simulink model "Model_TranslationEngine64"  (R2022b)
settings: Solver=FixedStepDiscrete  StartTime=0.0  StopTime=5  RelTol=1e-3  EnableMultiTasking=on
InitFcn:
  | % Initialize model
  | ModelSettings=BTConfig.GetModelSettings();
  | 
  | ModelSettings.Validate();
  | 
  | ModelInit;
  | 
  | 
  | % load library data
  | GainLibrary_data;
  | % Load saved values from partition process
  | CapturedConstMask.LoadMapFromFile(bdroot)
StartFcn:
  | % make sure all the simulated RTC requests are found
  | %RTC_SIM_OBJ.ValidateREQs();
undefined symbols (not defined in the file or in its folder): AA, BPLP, Column, NumHFRefBPF, NumHFRefLPF, NumMusicChannels, Row, VolumeMuteConfig
libraries: TuneVar x925, TOP x490, FeaturePath x111, CapturedConstLib x52
(part 30 of 34)

== matlab function Model_TranslationEngine64/ModelPreAmp/DecRate/Medusa5H1/SleepingBeauty/SleepingBeauty/Enabled/FadeControl/InnerLink/TuneVarFadeTable/Fade_Table_Translation ==
  data: tableDb output; fadeTable input; tableIdx output
  events: trigger input FUNCTION_CALL_EVENT
function [tableDb, tableIdx] = fcn(fadeTable)
%#codegen

% Set up the size and datatype of our TOP outputs:
maxTableSize = numel(fadeTable.Value) / 2;
idxType = 'uint8';
idxStorageType = 'uint32';
dbType = 'single';
tableIdx = zeros(1,maxTableSize,idxStorageType);
tableDb = zeros(1,maxTableSize,dbType);

% separate the pairs into their index and value components
givenPairs = fadeTable.Size(1);
indexes = fadeTable.Value(1:givenPairs,1);
values = fadeTable.Value(1:givenPairs,2);

% then sort and ignore duplicates
[cleanIdx,map] = unique(indexes);

% Validate input sizes
numPairs = numel(map);
argName='FadeTable';

% Validate: enough data?
if (numPairs < 2)
    TranslateError('%s must have at least 2 index pairs. Encounted value with only %f pairs\n', argName, numPairs);
end

% Validate: Highest index still below 1.0?
if (cleanIdx(1) < 0 || cleanIdx(end) > intmax(idxType))
    TranslateError('%s out of range table index %f encountered. Index must be between 0 and 255.\n',argName,cleanIdx(end));
end

% fill in the table buffer with provided pairs
tableIdx(1:numPairs) = cleanIdx(1:numPairs);
tableDb(1:numPairs) = values(map(1:numPairs));

% fill the rest of the table buffer with the last entry
remainingPairs = numel(map)+1:maxTableSize;
tableIdx(remainingPairs) = tableIdx(numPairs);
tableDb(remainingPairs) =  tableDb(numPairs);

end

== matlab function Model_TranslationEngine64/ModelPreAmp/DecRate/Medusa5H1/SleepingBeauty/SleepingBeauty/Enabled/FadeRamperDR/InnerLink/Channel_Ramper_Translation ==
  data: ChanRampMap output; TuneChanRampMap input; channelCount input; MaskNumChannelGroups parameter
  events: trigger input FUNCTION_CALL_EVENT
function ChanRampMap  = fcn(TuneChanRampMap, channelCount,... % inputs
    MaskNumChannelGroups) % parameters

% Verifies if each channel is assigned to either the 'Front'(1) or 'Rear'(2)
% groups. 

argName = 'Fade';

% Ensure each channel is present in the map
inputMapWidth = numel(TuneChanRampMap.Value);
if (inputMapWidth ~= channelCount)
   error(['Error in %s : Channel-to-ramper map width [%d] does not match number of ',...
       'audio channels [%d]. Make sure all channels are assigned ',...
       'to either the front or rear groups.'], argName, inputMapWidth, ...
       channelCount);
end

% Verify that the channels are assigned to valid group numbers
if (numel(unique(TuneChanRampMap.Value)) > MaskNumChannelGroups + 1)
    error(['Error in [%s] : Atleast 1 channel has been assigned to an incorrect group. ' ...
        'Group numbers assigned to channels in the Channel-to-ramper '...
        'map should either be ''1'' (Front), ''2'' (Rear), or ''-1'' (Unused).'], argName);        
end

% Ensure that a value of 0 was not entered as a ramper
if (sum(TuneChanRampMap.Value == 0) > 0)
   error(['Error in [%s] : Valid ramper values for the channel to '...
       'ramper map must be either 1, 2, or "-1" to indicate an '... 
       'unused channel .'], argName);
end

% Output
ChanRampMap = int32(TuneChanRampMap.Value);

== matlab function Model_TranslationEngine64/ModelPreAmp/DecRate/Medusa5H1/MedusaHoligram/Medusa5H1 Part 3/On/VLS Gains Computation/VLS Gains Pax/SLC Tuning/Detent Level/Trivial Translation ==
  data: TOP output; detentGain input; configStruct parameter
  events: trigger input FUNCTION_CALL_EVENT
function TOP  = fcn(detentGain, configStruct)
%#codegen

% Checks if the parameter satisfies dimensionality requirements
if(detentGain.Size(1) ~= configStruct.numGains)
    TranslateError('The parameter ''VLS_gains_detent'' must be a %d element vector.', configStruct.numGains);
end

% Checks if the parameter values follow bound requirements
checkValues = (detentGain.Value < 0);    
if(sum(sum(checkValues)))       % Results in 0 if all values in the matrix respect the bound requirements
    TranslateError('The weights in ''VLS_gains_detent'' must be greater than or equal to 0.');
end

TOP = detentGain.Value;

end

== matlab function Model_TranslationEngine64/ModelPreAmp/DecRate/Medusa5H1/MedusaHoligram/Medusa5H1 Part 3/On/VLS Gains Computation/VLS Gains Pax/SLC Tuning/Interpolation Method/Trivial Translation ==
  data: TOP output; interpolationMethod input
  events: trigger input FUNCTION_CALL_EVENT
function TOP  = fcn(interpolationMethod)
%#codegen
% Checks if the parameter satisfies dimensionality requirements
if(numel(interpolationMethod.Value) ~= 1)
   TranslateError('The parameter ''medusa_surround_db_interpolation'' must be single dimensional.'); 
end

% Checks if the parameter value follows bound requirements
if((interpolationMethod.Value ~= 0) && (interpolationMethod.Value ~= 1))
   TranslateError('The value of ''medusa_surround_db_interpolation'' must be either 0 (for linear interpolation) or 1 (for dB-linear interpolation).'); 
end

TOP = interpolationMethod.Value;

end

== matlab function Model_TranslationEngine64/ModelPreAmp/DecRate/Medusa5H1/MedusaHoligram/Medusa5H1 Part 3/On/VLS Gains Computation/VLS Gains Pax/SLC Tuning/Max Level/Trivial Translation ==
  data: TOP output; maxGain input; configStruct parameter
  events: trigger input FUNCTION_CALL_EVENT
function TOP  = fcn(maxGain, configStruct)
%#codegen

% Checks if the parameter satisfies dimensionality requirements
if(maxGain.Size(1) ~= configStruct.numGains)
    TranslateError('The parameter ''VLS_gains_max'' must be a %d element vector.', configStruct.numGains);
end

% Checks if the parameter values follow bound requirements
checkValues = (maxGain.Value < 0);
if(sum(sum(checkValues)))          % Results in 0 if all values in the matrix respect the bound requirements
    TranslateError('The weights in ''VLS_gains_max'' must be greater than or equal to 0.');
end

TOP = maxGain.Value;

end

== matlab function Model_TranslationEngine64/ModelPreAmp/DecRate/Medusa5H1/MedusaHoligram/Medusa5H1 Part 3/On/VLS Gains Computation/VLS Gains Pax/SLC Tuning/Min Level/Trivial Translation ==
  data: TOP output; minGain input; configStruct parameter
  events: trigger input FUNCTION_CALL_EVENT
function TOP  = fcn(minGain, configStruct)
%#codegen

% Checks if the parameter satisfies dimensionality requirements
if(minGain.Size(1) ~= configStruct.numGains)
    TranslateError('The parameter ''VLS_gains_min'' must be a %d element vector.', configStruct.numGains);
end

% Checks if the parameter values follow bound requirements
checkValues = (minGain.Value < 0);
if(sum(sum(checkValues)))          % Results in 0 if all values in the matrix respect the bound requirements
    TranslateError('The weights in ''VLS_gains_min'' must be greater than or equal to 0.');
end

TOP = minGain.Value;

end

== matlab function Model_TranslationEngine64/ModelPreAmp/DecRate/Medusa5H1/SleepingBeauty/SleepingBeauty/Enabled/FadeRamperDR/InnerLink/Filter_Coeffs_Translation ==
  data: FilterCoeffs output; cutoffFreqHz input; FsHz input
  events: trigger input FUNCTION_CALL_EVENT
function FilterCoeffs  = fcn(cutoffFreqHz, FsHz)

% Generate the low pass filter coefficients which will then be applied to
% the audio input
% Inputs:
%  cutoffFreqHz: Cut off frequency in Hz for LPF
%  FsHz: Sampling frequency in Hz

omega = 2 * pi * cutoffFreqHz.Value / FsHz;

A = 1 - sin(omega) / cos(omega);
B0 = (1 - A) / 2;
B1 = B0;

FilterCoeffs = single([B0 B1 A]);

== matlab function Model_TranslationEngine64/ModelPreAmp/DecRate/Medusa5H1/SleepingBeauty/SleepingBeauty/Enabled/FadeRamperFR/InnerLink/Channel_Ramper_Translation ==
  data: ChanRampMap output; TuneChanRampMap input; channelCount input; MaskNumChannelGroups parameter
  events: trigger input FUNCTION_CALL_EVENT
function ChanRampMap  = fcn(TuneChanRampMap, channelCount,... % inputs
    MaskNumChannelGroups) % parameters

% Verifies if each channel is assigned to either the 'Front'(1) or 'Rear'(2)
% groups. 

argName = 'Fade';

% Ensure each channel is present in the map
inputMapWidth = numel(TuneChanRampMap.Value);
if (inputMapWidth ~= channelCount)
   error(['Error in %s : Channel-to-ramper map width [%d] does not match number of ',...
       'audio channels [%d]. Make sure all channels are assigned ',...
       'to either the front or rear groups.'], argName, inputMapWidth, ...
       channelCount);
end

% Verify that the channels are assigned to valid group numbers
if (numel(unique(TuneChanRampMap.Value)) > MaskNumChannelGroups + 1)
    error(['Error in [%s] : Atleast 1 channel has been assigned to an incorrect group. ' ...
        'Group numbers assigned to channels in the Channel-to-ramper '...
        'map should either be ''1'' (Front), ''2'' (Rear), or ''-1'' (Unused).'], argName);        
end

% Ensure that a value of 0 was not entered as a ramper
if (sum(TuneChanRampMap.Value == 0) > 0)
   error(['Error in [%s] : Valid ramper values for the channel to '...
       'ramper map must be either 1, 2, or "-1" to indicate an '... 
       'unused channel .'], argName);
end

% Output
ChanRampMap = int32(TuneChanRampMap.Value);

== matlab function Model_TranslationEngine64/ModelPreAmp/DecRate/Medusa5H1/SleepingBeauty/SleepingBeauty/Enabled/FadeRamperFR/InnerLink/Filter_Coeffs_Translation ==
  data: FilterCoeffs output; cutoffFreqHz input; FsHz input
  events: trigger input FUNCTION_CALL_EVENT
function FilterCoeffs  = fcn(cutoffFreqHz, FsHz)

% Generate the low pass filter coefficients which will then be applied to
% the audio input
% Inputs:
%  cutoffFreqHz: Cut off frequency in Hz for LPF
%  FsHz: Sampling frequency in Hz

omega = 2 * pi * cutoffFreqHz.Value / FsHz;

A = 1 - sin(omega) / cos(omega);
B0 = (1 - A) / 2;
B1 = B0;

FilterCoeffs = single([B0 B1 A]);

== matlab function Model_TranslationEngine64/ModelPreAmp/DecRate/AudioPilot35/EntertainmentLevelDetection/AudiopilotLevelDetect/AudiopilotLevelDetect/HoldMargin/SetPositive ==
  data: TOP output single; Tune input
  events: trigger input FUNCTION_CALL_EVENT
function TOP = fcn(Tune)
%#codegen

TOP = abs(Tune.Value);

== matlab function Model_TranslationEngine64/ModelPreAmp/DecRate/Medusa5H1/SleepingBeauty/SleepingBeauty/Enabled/SleepingBeautyFR/InnerLink/TuneVarTable/translation ==
  data: tableDb output; sleepingBeautyTable input; tableIdx output
  events: trigger input FUNCTION_CALL_EVENT
function [tableDb, tableIdx]  = fcn(sleepingBeautyTable)
%#codegen

% Set up the size and datatype of our TOP outputs:
maxTableSize = numel(sleepingBeautyTable.Value) / 2;
idxType = 'uint8';
idxStorageType = 'uint32';
dbType = 'single';
tableIdx = zeros(1,maxTableSize,idxStorageType);
tableDb = zeros(1,maxTableSize,dbType);

% separate the pairs into their index and value components
givenPairs = sleepingBeautyTable.Size(1);
indices = sleepingBeautyTable.Value(1:givenPairs,1);
values = sleepingBeautyTable.Value(1:givenPairs,2);

% then sort and ignore duplicates
[cleanIdx,map] = unique(indices);

% Validate input sizes
numPairs = numel(map);
argName='sleepingBeautyTable';

% Validate: enough data?
if (numPairs < 2)
    TranslateError('%s must have at least 2 index pairs. Encounted value with only %f pairs\n', argName, numPairs);
end

% Validate: Highest index still below 255?
if (cleanIdx(1) < 0 || cleanIdx(end) > intmax(idxType))
    TranslateError('%s out of range table index %f encountered. Index must be between 0 and %d.\n',argName,cleanIdx(end),intmax(idxType));
end

% fill in the table buffer with provided pairs
tableIdx(1:numPairs) = cleanIdx(1:numPairs);
tableDb(1:numPairs) = values(map(1:numPairs));

% fill the rest of the table buffer with the last entry
remainingPairs = numel(map)+1:maxTableSize;
tableIdx(remainingPairs) = tableIdx(numPairs);
tableDb(remainingPairs) =  tableDb(numPairs);

end

== matlab function Model_TranslationEngine64/ModelPreAmp/DecRate/Medusa5H1/VLS/VLS Generation - D/translation ==
  data: FIRCoeffs output; FIRCoeffsIn input; PaddedFIRLengthsIn input; PaddedFIRLengths output
  events: trigger input FUNCTION_CALL_EVENT
function [FIRCoeffs, PaddedFIRLengths] = fcn(FIRCoeffsIn, PaddedFIRLengthsIn)

FIRCoeffs = FIRCoeffsIn.Value;
PaddedFIRLengths = PaddedFIRLengthsIn.Value;

== matlab function Model_TranslationEngine64/ModelPreAmp/DecRate/Medusa5H1/SleepingBeauty/SleepingBeauty/Enabled/SleepingBeautyDR/InnerLink/channel_ramper_translation ==
  data: ChanRampMap output; TuneChanRampMap input; channelCount input; MaskNumRampers parameter
  events: trigger input FUNCTION_CALL_EVENT
function ChanRampMap = fcn(TuneChanRampMap, channelCount, ... %Inputs
    MaskNumRampers) % Parameters

% Function that verifies channel-to-ramper map is valid
% Takes channelRamperMap and channelCount as inputs, and 
% number of rampers as a parameter
argName = 'SleepingBeauty';

% Ensure each channel is present in the map
inputMapWidth = numel(TuneChanRampMap.Value);
if (inputMapWidth ~= channelCount)
   error(['Error in %s : Channel-to-ramper map width [%d] does not match number of ',...
       'audio channels [%d]. Make sure all channels are assigned ',...
       'to either the left or right groups.'], argName, inputMapWidth, ...
       channelCount);
end

% Verifies if each channel is assigned to one of the 5 possible rampers.

if (numel(unique(TuneChanRampMap.Value)) > (MaskNumRampers + 1))
    error(['Error in [%s] : Atleast 1 channel has been assigned to the incorrect group.' ...
        'Group numbers assigned to channels in the Channel-to-ramper '...
        'map should be a number between 1 and [%d], corresponding to one '...
        'of the 3 possible speaker contents .'], argName, MaskNumRampers);        
end

% Verify that a value of 0 was not incorrectly entered as a ramper
if (sum(TuneChanRampMap.Value == 0) > 0)
   error(['Error in [%s] : Valid ramper values for the channel to '...
       'ramper map must be between 1 and [%d}, or "-1" to indicate an '... 
       'unused channel .'], argName), MaskNumRampers;
end

ChanRampMap = int32(TuneChanRampMap.Value);

== matlab function Model_TranslationEngine64/ModelPreAmp/DecRate/Medusa5H1/VLS/Crosstalk Cancellation/Pooliir with Non-Trivial Translations/InnerLink/PoolIirTunableWithReset/Translation ==
  data: RawSOS input; NumStages input; PoolNumStages output; PoolCoeffs output; MaxNumStages parameter; VariantUint8 parameter; NumChannels input
  events: trigger input FUNCTION_CALL_EVENT
function [PoolNumStages, PoolCoeffs] = pooliirTranslation(RawSOS, NumStages, MaxNumStages, VariantUint8,  NumChannels)
%#codegen

% Translation from raw SOS for pool SOS

% Some build time sanity size checking before calling the translation
if numel(NumStages.Value) ~= NumChannels
    error('Size of num stages has to match number of input channels')
end

if RawSOS.Size(2) ~= 6
    error ('Coefficient pool matrix must have 6 columns')
end

[PoolNumStages, PoolCoeffs] = poolIirTranslation(RawSOS, NumStages, MaxNumStages, VariantUint8);

% VariantStr = char(VariantUint8);
% switch (VariantStr)
%     case {"Generic","SharcPlusCore"}
%         % These variants order biquad coefficients in a compacted form
%         [PoolNumStages, PoolCoeffs] = pooliirTranslationFcn(RawSOS, NumStages, MaxNumStages);
%     case {"SharcPlusAccelGul","SharcPlusAccelGxp"}
%         % These variants order biquad coefficients for the ADI accelerator
%         [PoolNumStages, PoolCoeffs] = pooliirAccelTranslationFcn(RawSOS, NumStages, MaxNumStages);
%     case{"Hexagon"}
%         % Hexagon specific order for biquad coefficients 
%         [PoolNumStages, PoolCoeffs] = PoolIirHexagonTranslationFcn(RawSOS, NumStages, MaxNumStages);
%     case{"ArmNeonV7V8"}
%         [PoolNumStages, PoolCoeffs] = PoolIirArmNeonV7V8TranslationFcn(RawSOS, NumStages, MaxNumStages);
%     otherwise
%         % This is a build-time error, not a translation error. The
%         % selected build-time variant is not supported for translation
%         error('Invalid implementation type: [%s]', VariantStr);
% end

end

== matlab function Model_TranslationEngine64/ModelPreAmp/DecRate/Medusa5H1/SleepingBeauty/SleepingBeauty/Enabled/SleepingBeautyFR/InnerLink/channel_ramper_translation ==
  data: ChanRampMap output; TuneChanRampMap input; channelCount input; MaskNumRampers parameter
  events: trigger input FUNCTION_CALL_EVENT
function ChanRampMap = fcn(TuneChanRampMap, channelCount, ... %Inputs
    MaskNumRampers) % Parameters

% Function that verifies channel-to-ramper map is valid
% Takes channelRamperMap and channelCount as inputs, and 
% number of rampers as a parameter
argName = 'SleepingBeauty';

% Ensure each channel is present in the map
inputMapWidth = numel(TuneChanRampMap.Value);
if (inputMapWidth ~= channelCount)
   error(['Error in %s : Channel-to-ramper map width [%d] does not match number of ',...
       'audio channels [%d]. Make sure all channels are assigned ',...
       'to either the left or right groups.'], argName, inputMapWidth, ...
       channelCount);
end

% Verifies if each channel is assigned to one of the 5 possible rampers.

if (numel(unique(TuneChanRampMap.Value)) > (MaskNumRampers + 1))
    error(['Error in [%s] : Atleast 1 channel has been assigned to the incorrect group.' ...
        'Group numbers assigned to channels in the Channel-to-ramper '...
        'map should be a number between 1 and [%d], corresponding to one '...
        'of the 3 possible speaker contents .'], argName, MaskNumRampers);        
end

% Verify that a value of 0 was not incorrectly entered as a ramper
if (sum(TuneChanRampMap.Value == 0) > 0)
   error(['Error in [%s] : Valid ramper values for the channel to '...
       'ramper map must be between 1 and [%d}, or "-1" to indicate an '... 
       'unused channel .'], argName), MaskNumRampers;
end

ChanRampMap = int32(TuneChanRampMap.Value);

== matlab function Model_TranslationEngine64/ModelPreAmp/DecRate/Medusa5H1/VLS/VLS Generation - P/translation ==
  data: FIRCoeffs output; FIRCoeffsIn input; PaddedFIRLengthsIn input; PaddedFIRLengths output
  events: trigger input FUNCTION_CALL_EVENT
function [FIRCoeffs, PaddedFIRLengths] = fcn(FIRCoeffsIn, PaddedFIRLengthsIn)

FIRCoeffs = FIRCoeffsIn.Value;
PaddedFIRLengths = PaddedFIRLengthsIn.Value;

== matlab function Model_TranslationEngine64/ModelPreAmp/PreAmpPart1/NEARPreAmp/FixedAttenuator/Attenuation /Function-Call Subsystem/MATLAB Function ==
  data: dbgain input; lingain output
function lingain = fcn(dbgain)
    lingain = 10^(dbgain.Value/20);   
end

== matlab function Model_TranslationEngine64/NEAR/Near1p1/VolumeMute/AnnouncementLevelDetector/ch1_level/fast_decay/sec2samples ==
  data: y output; u input; FrameRate parameter
  events: trigger input FUNCTION_CALL_EVENT
function y  = fcn(u,FrameRate)
%#codegen

y = -abs(u.Value/FrameRate);

== matlab function Model_TranslationEngine64/ModelPreAmp/DecRate/Medusa5H1/SleepingBeauty/SleepingBeauty/Enabled/SleepingBeautyDR/InnerLink/TuneVarTable/translation ==
  data: tableDb output; sleepingBeautyTable input; tableIdx output
  events: trigger input FUNCTION_CALL_EVENT
function [tableDb, tableIdx]  = fcn(sleepingBeautyTable)
%#codegen

% Set up the size and datatype of our TOP outputs:
maxTableSize = numel(sleepingBeautyTable.Value) / 2;
idxType = 'uint8';
idxStorageType = 'uint32';
dbType = 'single';
tableIdx = zeros(1,maxTableSize,idxStorageType);
tableDb = zeros(1,maxTableSize,dbType);

% separate the pairs into their index and value components
givenPairs = sleepingBeautyTable.Size(1);
indices = sleepingBeautyTable.Value(1:givenPairs,1);
values = sleepingBeautyTable.Value(1:givenPairs,2);

% then sort and ignore duplicates
[cleanIdx,map] = unique(indices);

% Validate input sizes
numPairs = numel(map);
argName='sleepingBeautyTable';

% Validate: enough data?
if (numPairs < 2)
    TranslateError('%s must have at least 2 index pairs. Encounted value with only %f pairs\n', argName, numPairs);
end

% Validate: Highest index still below 255?
if (cleanIdx(1) < 0 || cleanIdx(end) > intmax(idxType))
    TranslateError('%s out of range table index %f encountered. Index must be between 0 and %d.\n',argName,cleanIdx(end),intmax(idxType));
end

% fill in the table buffer with provided pairs
tableIdx(1:numPairs) = cleanIdx(1:numPairs);
tableDb(1:numPairs) = values(map(1:numPairs));

% fill the rest of the table buffer with the last entry
remainingPairs = numel(map)+1:maxTableSize;
tableIdx(remainingPairs) = tableIdx(numPairs);
tableDb(remainingPairs) =  tableDb(numPairs);

end

== matlab function Model_TranslationEngine64/NEAR/Near1p1/VolumeMute/AnnouncementLevelDetector/ch1_level/hold_margin/SetPositive ==
  data: TOP output single; Tune input
  events: trigger input FUNCTION_CALL_EVENT
function TOP = fcn(Tune)
%#codegen

TOP = abs(Tune.Value);

== matlab function Model_TranslationEngine64/ModelPreAmp/PreAmpPart1/NEARPreAmp/MusicLimiter/annPredTuneTOP/Trivial Translation ==
  data: TOP1 output; Tune1 input
  events: trigger input FUNCTION_CALL_EVENT
function TOP1  = fcn(Tune1)
%#codegen

% ----- To access TuneVar maximum size, current size, and current value:
%   Note: TuneVar signals arrive with exposed variable size information.
%         The expressions below illustrate for the "Tune1" input argument.
%
%   size(Tune1.Value) : the maximum possible size of the Tune1 variable
%
%   Tune.Size   : the current size of *valid* data in Tune1.Value
%
%   Tune1.Size(1) : Number of rows present in Tune1 - this does not vary.
%
%   Tune1.Size(2) : Number of columns currently valid in Tune1 - this is
%       the variable part of size that can change (if allowed by TuneVar).
%
%   Tune1.Value : the current value of the tune variable... but end-padded 
%       to the maximum available size with undefined/invalid data.
%
%   numel(Tune1.Value) : another way of looking at the maximum number of
%       elements that could arrive in Tune1.Value
%
% ----- To register an error, use the following method (works like printf):
%   TranslateError( <format string>, <arguments ... )
%   ... this error will cause the build process to abort.

% A trivial pass-through translation looks like this:
%TOP1 = Tune1.Value;
TOP1 = 10 ^ ((Tune1.Value) / 20);

== matlab function Model_TranslationEngine64/NEAR/Near1p1/VolumeMute/AnnouncementLevelDetector/ch1_level/hold_time/sec2samples ==
  data: y output; u input; FrameRate parameter
  events: trigger input FUNCTION_CALL_EVENT
function y  = fcn(u,FrameRate)
%#codegen

y = ceil(u.Value*FrameRate);

== matlab function Model_TranslationEngine64/ModelPreAmp/PreAmpPart1/Bass/tone filter tune translate1 ==
  data: FilterCoeffs output; FilterFrequencyHz input; Fs input; MaskFilterType parameter
  events: trigger input FUNCTION_CALL_EVENT
function FilterCoeffs  = fcn( ...
    FilterFrequencyHz, Fs, ... % inputs
    MaskFilterType ) % parameters
%#codegen

omega = 2 * pi * FilterFrequencyHz.Value / Fs;

A = (1 - sin(omega)) / cos(omega);

if (MaskFilterType == ToneMask.TypeLowpass)
    % lowpass coeffs (e.g. bass)
    B0 = (1 - A) / 2;
    B1 = B0;
else
    % highpass coeffs (e.g. treble)
    B0 = (1 + A) / 2;
    B1 = 0 - B0;
end

FilterCoeffs = single([B0 B1 A]);

== matlab function Model_TranslationEngine64/ModelPreAmp/PreAmpPart1/Bass/tone filter tune translate2 ==
  data: FilterCoeffs output; FilterFrequencyHz input; Fs input; MaskFilterType parameter
  events: trigger input FUNCTION_CALL_EVENT
function FilterCoeffs  = fcn( ...
    FilterFrequencyHz, Fs, ... % inputs
    MaskFilterType ) % parameters
%#codegen

omega = 2 * pi * FilterFrequencyHz.Value / Fs;

A = (1 - sin(omega)) / cos(omega);

if (MaskFilterType == ToneMask.TypeLowpass)
    % lowpass coeffs (e.g. bass)
    B0 = (1 - A) / 2;
    B1 = B0;
else
    % highpass coeffs (e.g. treble)
    B0 = (1 + A) / 2;
    B1 = 0 - B0;
end

FilterCoeffs = single([B0 B1 A]);

== matlab function Model_TranslationEngine64/ModelPreAmp/PreAmpPart1/Bass/tone filter tune translate3 ==
  data: maxOut output; maxIn input
  events: trigger input FUNCTION_CALL_EVENT
function maxOut  = fcn( ...
    maxIn) ... % inputs % parameters
%#codegen

% Just make sure the maximum is a positive dB value
maxOut = single(abs(maxIn.Value));

== matlab function Model_TranslationEngine64/ModelPreAmp/PreAmpPart1/Bass/tone filter tune translate4 ==
  data: maxOut output; maxIn input
  events: trigger input FUNCTION_CALL_EVENT
function maxOut  = fcn( ...
    maxIn) ... % inputs % parameters
%#codegen

% Just make sure the maximum is a positive dB value
maxOut = single(abs(maxIn.Value));

== matlab function Model_TranslationEngine64/ModelPreAmp/PreAmpPart1/Midrange/tone filter tune translate1 ==
  data: FilterFrequencyHz input; Fs input; Qval input; FilterCoeffs output
  events: trigger input FUNCTION_CALL_EVENT
function FilterCoeffs  = fcn(FilterFrequencyHz, Fs, Qval)
%#codegen
% Compute the discrete frequency
omega = 2 * pi * FilterFrequencyHz.Value / Fs;
Q = Qval.Value;

% Equations for computing filter coefficients of a bandpass filter
% Compute the denominator coeffs
A1 = (-4 * Q * cos(omega)) / (2 * Q + sin(omega));
A2 = (2 * Q - sin(omega)) / (2 * Q + sin(omega));
% Compute the numerator coeffs
B0 = sin(omega)/ (2 * Q + sin(omega));
B1 = 0;
B2 = -B0;
% Concatenate to obtain the final coeffs
FilterCoeffs = single([A1 A2 B0 B1 B2]);

== matlab function Model_TranslationEngine64/ModelPreAmp/PreAmpPart1/Midrange/tone filter tune translate2 ==
  data: FilterFrequencyHz input; Fs input; Qval input; FilterCoeffs output
  events: trigger input FUNCTION_CALL_EVENT
function FilterCoeffs  = fcn(FilterFrequencyHz, Fs, Qval)
%#codegen
% Compute the discrete frequency
omega = 2 * pi * FilterFrequencyHz.Value / Fs;
Q = Qval.Value;

% Equations for computing filter coefficients of a bandpass filter
% Compute the denominator coeffs
A1 = (-4 * Q * cos(omega)) / (2 * Q + sin(omega));
A2 = (2 * Q - sin(omega)) / (2 * Q + sin(omega));
% Compute the numerator coeffs
B0 = sin(omega)/ (2 * Q + sin(omega));
B1 = 0;
B2 = -B0;
% Concatenate to obtain the final coeffs
FilterCoeffs = single([A1 A2 B0 B1 B2]);

== matlab function Model_TranslationEngine64/ModelPreAmp/PreAmpPart1/Midrange/tone filter tune translate3 ==
  data: maxOut output; maxIn input
  events: trigger input FUNCTION_CALL_EVENT
function maxOut  = fcn( ...
    maxIn) ... % inputs % parameters
%#codegen

% Just make sure the maximum is a positive dB value
maxOut = single(abs(maxIn.Value));

== matlab function Model_TranslationEngine64/ModelPreAmp/DecRate/AudioPilot35/Audiopilot_3_5/ConfigurationRtcInputs/Hvac/table/TableFormatting ==
  data: tableTOP output; table input; MaskHvacTableSize parameter
  events: trigger input FUNCTION_CALL_EVENT
function tableTOP  = fcn(table, MaskHvacTableSize)
    %#codegen

    % "table": Table containing noise values corresponding to different HVAC
    % settings. Column 1 contains the 'HVAC Setting' and varies from
    % [0,1.0]. Column 2 contains the corresponding 'HVAC noise' values.
    % Error checks for the HVAC table:
    % 1. Column1 must have atleast 2 unique values.
    % 2. Each unique value in column 1 can correspond to only one noise value.
    %    Example- An HVAC setting of 0.5 cannot correspond to both 60 dBSPL and 70 dBSPL.
    % 3. If there are duplicate pairs in the table, only one is retained.
    % 4. Column2 values are expected to either increase with an increase in HVAC setting or remain constant.
    %    Example - The noise corresponding to an HVAC setting of 1.0 must be 
    %    higher than or equal to that of 0.5.
    % 5. If the table does not contain the entries for HVAC settings 0.0 or
    %    1.0, they are added in the translation so that the interpolation
    %    can handle any incoming control messages in the range [0.0, 1.0].
    %    Example - [0.5,70 ; 
    % 6. Size restrictions - the table must have 2 columns and <= MaskHvacTableSize rows.    
    
    % "tableTOP": Output table [16x2] after performing checks

    argName = 'AudioPilot 3.5 HVAC';
    tableTOP = zeros(MaskHvacTableSize,2,'single');
    numEntries = table.Size(1);
    table = table.Value(1:numEntries,:);

    % Sort the table with respect to the fan setting (ascending). 
    % Ensure that the corresponding noise values are also in the ascending 
    % order by checking if the difference between consecutive elements is 
    % always non negative.
    table = sortrows(table,1);
    isNoiseIncreasing = all(diff(table(:,2)) >= 0);
    if ~isNoiseIncreasing
        TranslateError('Error in %s: Noise values must increase with increase in fan current.',argName);
    end
    
    % Ensure that the lowest fan setting is 0 and the highest is 1.0 for
    % the interpolation to work. Using an intermediate variable to add the
    % new row.
    if table(1,1) ~= single(0.0)
        numRows = size(table,1) + 1;
        updatedTable = zeros(numRows,2,'single');
        updatedTable(1,1) = 0.0;
        updatedTable(1,2) = table(1,2);
        updatedTable(2:numRows,:) = table;
        table = updatedTable;
    end
    if table(end,1) ~= single(1.0)
        numRows = size(table,1) + 1;
        updatedTable = zeros(numRows,2,'single');
        updatedTable(numRows,1) = 1.0;
        updatedTable(numRows,2) = table(numRows-1,2);
        updatedTable(1:numRows-1,:) = table;
        table = updatedTable;
    end
    fanSetting = table(:,1);
    noise = table(:,2);
    numEntries = numel(fanSetting);
    
    % Check for unique indexes in fan settings. If a fan setting has a
    % duplicate, check if the corresponding noise values are the same. If
    % they are the same, then only one pair is retained and the others
    % discarded. If they are different, an error is thrown as one fan
    % setting cannot correspond to multiple noise values.
    [fanSettingUnique,idxUnique] = unique(fanSetting);
    duplicateIdx = setdiff(1:numEntries,idxUnique);
    
    for i = 1:numel(duplicateIdx)
        currFanSetting = fanSetting(duplicateIdx(i));
        dupNoise = noise( fanSetting == currFanSetting );
        IsCorrespondingNoiseEqual = all(dupNoise == dupNoise(1));
        if IsCorrespondingNoiseEqual ~= 1
            TranslateError('Error in %s: Fan settings [%f] corresponds to multiple noise values. Ensure that each fan setting corresponds only to one noise value.',argName,currFanSetting);
        end
    end 
    
    numEntriesUnique = numel(fanSettingUnique);
    noiseUnique = noise(idxUnique);
    
    % Number of table entries needs to be atleast 2 for the interp1 function to
    % work and less than equal to MaskHvacTableSize. The fan setting can
    % only be in the range [0,1.0].
    if (numEntriesUnique < 2)
        TranslateError('Error in %s: Noise table must have atleast 2 unique fan settings.',argName);
    end
    if (numEntriesUnique > MaskHvacTableSize)
        TranslateError('Error in %s: Noise table cannot be longer than [%d].', argName,MaskHvacTableSize);
    end
    if (any(fanSetting > 1) || any(fanSetting < 0))
        TranslateError('Error in %s: Fan setting needs to be between 0 and 1.', argName);
    end
    
    % Create the output TOP matrix 
    tableTOP(1:numEntriesUnique,1) = fanSettingUnique;
    tableTOP(1:numEntriesUnique,2) = noiseUnique;
    
end

== matlab function Model_TranslationEngine64/ModelPreAmp/PreAmpPart1/Midrange/tone filter tune translate4 ==
  data: maxOut output; maxIn input
  events: trigger input FUNCTION_CALL_EVENT
function maxOut  = fcn( ...
    maxIn) ... % inputs % parameters
%#codegen

% Just make sure the maximum is a positive dB value
maxOut = single(abs(maxIn.Value));

== matlab function Model_TranslationEngine64/NEAR/Near1p1/VolumeMute/AnnouncementLevelDetector/ch1_level/slow_decay/sec2samples ==
  data: y output; u input; FrameRate parameter
  events: trigger input FUNCTION_CALL_EVENT
function y  = fcn(u,FrameRate)
%#codegen

y = -abs(u.Value/FrameRate);

== matlab function Model_TranslationEngine64/ModelPreAmp/PreAmpPart1/NEARPreAmp/MusicLimiter/limiter/MATLAB Function2 ==
  data: u input; y output; Fs input
  events: trigger input FUNCTION_CALL_EVENT
function y = fcn(u, Fs)

y = single(undb20(abs(u.Value) / Fs));

== matlab function Model_TranslationEngine64/ModelPreAmp/PreAmpPart1/NEARPreAmp/MusicLimiter/limiter/MATLAB Function3 ==
  data: attackDB input; Fs input; attack output
  events: trigger input FUNCTION_CALL_EVENT
%function [attack, k1]= fcn(attackDB, threshold, Fs)
function attack = fcn(attackDB, Fs)
attack = single(1 - undb20(-abs(attackDB.Value) / Fs));
%k1 = attack ./ single(threshold.Value);

== matlab function Model_TranslationEngine64/ModelPreAmp/PreAmpPart1/NEARPreAmp/MusicLimiter/limiter/MATLAB Function4 ==
  data: u input; y output
  events: trigger input FUNCTION_CALL_EVENT
function y = fcn(u)

y = single(undb20(-abs(u.Value)));

== matlab function Model_TranslationEngine64/ModelPreAmp/PreAmpPart1/NEARPreAmp/MusicLimiter/offsetTuneTOP/Trivial Translation ==
  data: TOP1 output; Tune1 input
  events: trigger input FUNCTION_CALL_EVENT
function TOP1  = fcn(Tune1)
%#codegen

% ----- To access TuneVar maximum size, current size, and current value:
%   Note: TuneVar signals arrive with exposed variable size information.
%         The expressions below illustrate for the "Tune1" input argument.
%
%   size(Tune1.Value) : the maximum possible size of the Tune1 variable
%
%   Tune.Size   : the current size of *valid* data in Tune1.Value
%
%   Tune1.Size(1) : Number of rows present in Tune1 - this does not vary.
%
%   Tune1.Size(2) : Number of columns currently valid in Tune1 - this is
%       the variable part of size that can change (if allowed by TuneVar).
%
%   Tune1.Value : the current value of the tune variable... but end-padded 
%       to the maximum available size with undefined/invalid data.
%
%   numel(Tune1.Value) : another way of looking at the maximum number of
%       elements that could arrive in Tune1.Value
%
% ----- To register an error, use the following method (works like printf):
%   TranslateError( <format string>, <arguments ... )
%   ... this error will cause the build process to abort.

% A trivial pass-through translation looks like this:
%TOP1 = Tune1.Value;
TOP1 = 10 ^ ((Tune1.Value) / 20);

== matlab function Model_TranslationEngine64/ModelPreAmp/PreAmpPart1/NEARPreAmp/MusicLimiter/upperThresholdTuneTOP/Trivial Translation ==
  data: TOP1 output; Tune1 input
  events: trigger input FUNCTION_CALL_EVENT
function TOP1  = fcn(Tune1)
%#codegen

% ----- To access TuneVar maximum size, current size, and current value:
%   Note: TuneVar signals arrive with exposed variable size information.
%         The expressions below illustrate for the "Tune1" input argument.
%
%   size(Tune1.Value) : the maximum possible size of the Tune1 variable
%
%   Tune.Size   : the current size of *valid* data in Tune1.Value
%
%   Tune1.Size(1) : Number of rows present in Tune1 - this does not vary.
%
%   Tune1.Size(2) : Number of columns currently valid in Tune1 - this is
%       the variable part of size that can change (if allowed by TuneVar).
%
%   Tune1.Value : the current value of the tune variable... but end-padded 
%       to the maximum available size with undefined/invalid data.
%
%   numel(Tune1.Value) : another way of looking at the maximum number of
%       elements that could arrive in Tune1.Value
%
% ----- To register an error, use the following method (works like printf):
%   TranslateError( <format string>, <arguments ... )
%   ... this error will cause the build process to abort.

% A trivial pass-through translation looks like this:
%TOP1 = Tune1.Value;
TOP1 = 10 ^ ((Tune1.Value) / 20);

== matlab function Model_TranslationEngine64/NEAR/Near1p1/VolumeMute/AnnouncementLevelDetector/ch2_level/fast_decay/sec2samples ==
  data: y output; u input; FrameRate parameter
  events: trigger input FUNCTION_CALL_EVENT
function y  = fcn(u,FrameRate)
%#codegen

y = -abs(u.Value/FrameRate);

== matlab function Model_TranslationEngine64/ModelPreAmp/PreAmpPart1/Treble/tone filter tune translate1 ==
  data: FilterCoeffs output; FilterFrequencyHz input; Fs input; MaskFilterType parameter
  events: trigger input FUNCTION_CALL_EVENT
function FilterCoeffs  = fcn( ...
    FilterFrequencyHz, Fs, ... % inputs
    MaskFilterType ) % parameters
%#codegen

omega = 2 * pi * FilterFrequencyHz.Value / Fs;

A = (1 - sin(omega)) / cos(omega);

if (MaskFilterType == ToneMask.TypeLowpass)
    % lowpass coeffs (e.g. bass)
    B0 = (1 - A) / 2;
    B1 = B0;
else
    % highpass coeffs (e.g. treble)
    B0 = (1 + A) / 2;
    B1 = 0 - B0;
end

FilterCoeffs = single([B0 B1 A]);

== matlab function Model_TranslationEngine64/ModelPreAmp/PreAmpPart1/Treble/tone filter tune translate2 ==
  data: FilterCoeffs output; FilterFrequencyHz input; Fs input; MaskFilterType parameter
  events: trigger input FUNCTION_CALL_EVENT
function FilterCoeffs  = fcn( ...
    FilterFrequencyHz, Fs, ... % inputs
    MaskFilterType ) % parameters
%#codegen

omega = 2 * pi * FilterFrequencyHz.Value / Fs;

A = (1 - sin(omega)) / cos(omega);

if (MaskFilterType == ToneMask.TypeLowpass)
    % lowpass coeffs (e.g. bass)
    B0 = (1 - A) / 2;
    B1 = B0;
else
    % highpass coeffs (e.g. treble)
    B0 = (1 + A) / 2;
    B1 = 0 - B0;
end

FilterCoeffs = single([B0 B1 A]);

== matlab function Model_TranslationEngine64/ModelPreAmp/DecRate/AudioPilot35/EntertainmentLevelDetection/AudiopilotLevelDetect/AudiopilotLevelDetect/HoldTime/sec2samples ==
  data: y output; u input; FrameRate parameter
  events: trigger input FUNCTION_CALL_EVENT
function y  = fcn(u,FrameRate)
%#codegen

y = ceil(u.Value*FrameRate);

== matlab function Model_TranslationEngine64/ModelPreAmp/PreAmpPart1/Treble/tone filter tune translate3 ==
  data: maxOut output; maxIn input
  events: trigger input FUNCTION_CALL_EVENT
function maxOut  = fcn( ...
    maxIn) ... % inputs % parameters
%#codegen

% Just make sure the maximum is a positive dB value
maxOut = single(abs(maxIn.Value));

== matlab function Model_TranslationEngine64/ModelPreAmp/PreAmpPart1/Treble/tone filter tune translate4 ==
  data: maxOut output; maxIn input
  events: trigger input FUNCTION_CALL_EVENT
function maxOut  = fcn( ...
    maxIn) ... % inputs % parameters
%#codegen

% Just make sure the maximum is a positive dB value
maxOut = single(abs(maxIn.Value));

== matlab function Model_TranslationEngine64/NEAR/Near1p1/VolumeMute/AnnouncementLevelDetector/ch2_level/hold_margin/SetPositive ==
  data: TOP output single; Tune input
  events: trigger input FUNCTION_CALL_EVENT
function TOP = fcn(Tune)
%#codegen

TOP = abs(Tune.Value);

== matlab function Model_TranslationEngine64/NEAR/Near1p1/DrProc/FsEQDr/Subsystem1/Translation ==
  data: eqdelays output single; F1 input; F2 input; F3 input; F4 input; F5 input; F6 input; F7 input
  events: trigger input FUNCTION_CALL_EVENT
function eqdelays  = fcn(   F1,...
                            F2,...
                            F3,...
                            F4,...
                            F5,...
                            F6,...
                            F7)
                   
eqdelays = single([ F1.Value,...
                        F2.Value,...
                        F3.Value,...
                        F4.Value,...
                        F5.Value,...
                        F6.Value,...
                        F7.Value]);
end

== matlab function Model_TranslationEngine64/NEAR/Near1p1/DrProc/FsEQDr/Pooliir/PoolIirTunableWithReset/Translation ==
  data: RawSOS input; NumStages input; PoolNumStages output; PoolCoeffs output; MaxNumStages parameter; VariantUint8 parameter; NumChannels input
  events: trigger input FUNCTION_CALL_EVENT
function [PoolNumStages, PoolCoeffs] = pooliirTranslation(RawSOS, NumStages, MaxNumStages, VariantUint8,  NumChannels)
%#codegen

% Translation from raw SOS for pool SOS

% Some build time sanity size checking before calling the translation
if numel(NumStages.Value) ~= NumChannels
    error('Size of num stages has to match number of input channels')
end

if RawSOS.Size(2) ~= 6
    error ('Coefficient pool matrix must have 6 columns')
end

[PoolNumStages, PoolCoeffs] = poolIirTranslation(RawSOS, NumStages, MaxNumStages, VariantUint8);

% VariantStr = char(VariantUint8);
% switch (VariantStr)
%     case {"Generic","SharcPlusCore"}
%         % These variants order biquad coefficients in a compacted form
%         [PoolNumStages, PoolCoeffs] = pooliirTranslationFcn(RawSOS, NumStages, MaxNumStages);
%     case {"SharcPlusAccelGul","SharcPlusAccelGxp"}
%         % These variants order biquad coefficients for the ADI accelerator
%         [PoolNumStages, PoolCoeffs] = pooliirAccelTranslationFcn(RawSOS, NumStages, MaxNumStages);
%     case{"Hexagon"}
%         % Hexagon specific order for biquad coefficients 
%         [PoolNumStages, PoolCoeffs] = PoolIirHexagonTranslationFcn(RawSOS, NumStages, MaxNumStages);
%     case{"ArmNeonV7V8"}
%         [PoolNumStages, PoolCoeffs] = PoolIirArmNeonV7V8TranslationFcn(RawSOS, NumStages, MaxNumStages);
%     otherwise
%         % This is a build-time error, not a translation error. The
%         % selected build-time variant is not supported for translation
%         error('Invalid implementation type: [%s]', VariantStr);
% end

end

== matlab function Model_TranslationEngine64/NEAR/Near1p1/DrProc/HrEQDr/Subsystem2/Translation ==
  data: eqdelays output single; driversrc1 input; driversrc2 input; driversrc3 input; driversrc4 input; passengersrc1 input; passengersrc2 input; passengersrc3 input; passengersrc4 input; NumHeadrestSpeakers parameter; AnnChannelCount parameter
  events: trigger input FUNCTION_CALL_EVENT
function eqdelays  = fcn(driversrc1, driversrc2, driversrc3, driversrc4, passengersrc1, passengersrc2, passengersrc3, passengersrc4, NumHeadrestSpeakers, AnnChannelCount)
    switch NumHeadrestSpeakers
        case 1
            switch AnnChannelCount
                case 1
                    eqdelays = single([driversrc1.Value, driversrc2.Value]);
                case 2
                    eqdelays = single([driversrc1.Value, driversrc2.Value]);
                case 3
                    eqdelays = single([driversrc1.Value, driversrc2.Value, driversrc3.Value]);
                case 4
                    eqdelays = single([driversrc1.Value, driversrc2.Value, driversrc3.Value, driversrc4.Value]);
            end
        case 2
            switch AnnChannelCount
                case 1
                    eqdelays = single([driversrc1.Value, driversrc2.Value, passengersrc1.Value, passengersrc2.Value]);
                case 2
                    eqdelays = single([driversrc1.Value, driversrc2.Value, passengersrc1.Value, passengersrc2.Value]);
                case 3
                    eqdelays = single([driversrc1.Value, driversrc2.Value, driversrc3.Value, passengersrc1.Value, passengersrc2.Value, passengersrc3.Value]);
                case 4
                    eqdelays = single([driversrc1.Value, driversrc2.Value, driversrc3.Value, driversrc4.Value, passengersrc1.Value, passengersrc2.Value, passengersrc3.Value, passengersrc4.Value]);
            end
    end

end

== matlab function Model_TranslationEngine64/NEAR/Near1p1/DrProc/HrEQDr/PoolIirTunable/PoolIirTunableWithReset/Translation ==
  data: RawSOS input; NumStages input; PoolNumStages output; PoolCoeffs output; MaxNumStages parameter; VariantUint8 parameter; NumChannels input
  events: trigger input FUNCTION_CALL_EVENT
function [PoolNumStages, PoolCoeffs] = pooliirTranslation(RawSOS, NumStages, MaxNumStages, VariantUint8,  NumChannels)
%#codegen

% Translation from raw SOS for pool SOS

% Some build time sanity size checking before calling the translation
if numel(NumStages.Value) ~= NumChannels
    error('Size of num stages has to match number of input channels')
end

if RawSOS.Size(2) ~= 6
    error ('Coefficient pool matrix must have 6 columns')
end

[PoolNumStages, PoolCoeffs] = poolIirTranslation(RawSOS, NumStages, MaxNumStages, VariantUint8);

% VariantStr = char(VariantUint8);
% switch (VariantStr)
%     case {"Generic","SharcPlusCore"}
%         % These variants order biquad coefficients in a compacted form
%         [PoolNumStages, PoolCoeffs] = pooliirTranslationFcn(RawSOS, NumStages, MaxNumStages);
%     case {"SharcPlusAccelGul","SharcPlusAccelGxp"}
%         % These variants order biquad coefficients for the ADI accelerator
%         [PoolNumStages, PoolCoeffs] = pooliirAccelTranslationFcn(RawSOS, NumStages, MaxNumStages);
%     case{"Hexagon"}
%         % Hexagon specific order for biquad coefficients 
%         [PoolNumStages, PoolCoeffs] = PoolIirHexagonTranslationFcn(RawSOS, NumStages, MaxNumStages);
%     case{"ArmNeonV7V8"}
%         [PoolNumStages, PoolCoeffs] = PoolIirArmNeonV7V8TranslationFcn(RawSOS, NumStages, MaxNumStages);
%     otherwise
%         % This is a build-time error, not a translation error. The
%         % selected build-time variant is not supported for translation
%         error('Invalid implementation type: [%s]', VariantStr);
% end

end

== matlab function Model_TranslationEngine64/NEAR/Near1p1/FrProc/Subsystem/FsEQFr/Subsystem1/Translation ==
  data: eqdelays output single; F1 input; F2 input; F3 input; F4 input; F5 input; F6 input; F7 input
  events: trigger input FUNCTION_CALL_EVENT
function eqdelays  = fcn(   F1,...
                            F2,...
                            F3,...
                            F4,...
                            F5,...
                            F6,...
                            F7)
                   
eqdelays = single([ F1.Value,...
                        F2.Value,...
                        F3.Value,...
                        F4.Value,...
                        F5.Value,...
                        F6.Value,...
                        F7.Value]);
end

== matlab function Model_TranslationEngine64/ModelPreAmp/DecRate/AudioPilot35/Audiopilot_3_5/GainApplication/Compensation/BassBpf/wcQ2coefs ==
  data: num output; freq input; Qin input; denom output; SampleRate parameter
  events: trigger input FUNCTION_CALL_EVENT
function [num,denom] = fcn(freq,Qin,SampleRate)
% Forms the numerator and denominator coefficients
% for a second-order band-pass filter with 
% the specified cutoff frequency and Q value

%#codegen


Fc = freq.Value;
Q = Qin.Value;

% The frequency in radians
wc = 2 * pi * Fc / SampleRate;
sinCoef = sin(wc);
cosCoef = cos(wc);

sos = [0 0 0];
sos(1) = (2*Q - sinCoef)/(2*Q + sinCoef);
sos(2) = -4*Q*cosCoef/(2*Q + sinCoef);
sos(3) = sinCoef/(2*Q + sinCoef);

num = sos(3)*[1 0 -1];
denom = [1 sos(2) sos(1)];
